simulink model "state_machine"  (R2012b)
settings: Solver=ode45  StartTime=0.0  StopTime=10.0  RelTol=1e-3
settings Model: Creator=h3now  LastModifiedBy=h3now

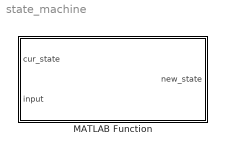
== system state_machine ==
  MATLAB Function : MATLAB Function  TreatAsAtomicUnit=on

== matlab function state_machine/MATLAB Function ==
  data: cur_state input; new_state output; input input
function new_state = state_machine(cur_state, input)
%#codegen

% Initializing persistent variable to store the angular position value.
persistent theta;
if isempty(theta)
    theta = 9;
end

% State machine.
switch cur_state
    case 0
        % keep state.
        if isequal(input,[0,0,0])
            new_state = cur_state;
        % go to next state.
        elseif isequal(input,[0,0,0])
            new_state = 1;
            theta = theta + 1;
        % go to previous state.
        elseif isequal(input,[0,0,0])
            new_state = 7;
            theta = theta - 1;
        % go to error state.
        else
            new_state = -1;
        end
        
    case 1
        % keep state.
        if isequal(input,[0,0,0])
            new_state = cur_state;
        % go to next state.
        elseif isequal(input,[0,0,0])
            new_state = 2;
            theta = theta + 1;
        % go to previous state.
        elseif isequal(input,[0,0,0])
            new_state = 0;
            theta = theta - 1;
        % go to error state.
        else
            new_state = -1;
        end
        
    case 2
        % keep state.
        if isequal(input,[0,0,0])
            new_state = cur_state;
        % go to next state.
        elseif isequal(input,[0,0,0])
            new_state = 3;
            theta = theta + 1;
        % go to previous state.
        elseif isequal(input,[0,0,0])
            new_state = 1;
            theta = theta - 1;
        % go to error state.
        else
            new_state = -1;
        end
        
    case 3
        % keep state.
        if isequal(input,[0,0,0])
            new_state = cur_state;
        % go to next state.
        elseif isequal(input,[0,0,0])
            new_state = 4;
            theta = theta + 1;
        % go to previous state.
        elseif isequal(input,[0,0,0])
            new_state = 2;
            theta = theta - 1;
        % go to error state.
        else
            new_state = -1;
        end
        
    case 4
        % keep state.
        if isequal(input,[0,0,0])
            new_state = cur_state;
        % go to next state.
        elseif isequal(input,[0,0,0])
            new_state = 5;
            theta = theta + 1;
        % go to previous state.
        elseif isequal(input,[0,0,0])
            new_state = 3;
            theta = theta - 1;
        % go to error state.
        else
            new_state = -1;
        end
        
    case 5
        % keep state.
        if isequal(input,[0,0,0])
            new_state = cur_state;
        % go to next state.
        elseif isequal(input,[0,0,0])
            new_state = 6;
            theta = theta + 1;
        % go to previous state.
        elseif isequal(input,[0,0,0])
            new_state = 4;
            theta = theta - 1;
        % go to error state.
        else
            new_state = -1;
        end
        
    case 6
        % keep state.
        if isequal(input,[0,0,0])
            new_state = cur_state;
        % go to next state.
        elseif isequal(input,[0,0,0])
            new_state = 7;
            theta = theta + 1;
        % go to previous state.
        elseif isequal(input,[0,0,0])
            new_state = 5;
            theta = theta - 1;
        % go to error state.
        else
            new_state = -1;
        end
        
    case 7
        % keep state.
        if isequal(input,[0,0,0])
            new_state = cur_state;
        % go to next state.
        elseif isequal(input,[0,0,0])
            new_state = 0;
            theta = theta + 1;
        % go to previous state.
        elseif isequal(input,[0,0,0])
            new_state = 6;
            theta = theta - 1;
        % go to error state.
        else
            new_state = -1;
        end     
end
